simulink model "Week2_pr2"  (R2020b)
settings: Solver=VariableStepAuto  StartTime=0.0  StopTime=10.0  RelTol=1e-3
model workspace (MAT data in the model file):
  Be = 2
  Bv = 1
  Fn = [0  0; 1  0.8; 2  1.6; 3  1.6; 4  1.6; 5  1.6; 6  0.8; 7  0; 8  0; 9  0; 10  0]
  Ie = 1
  Iv = 5
  Muk = 1
  Mus = 1.5
  R = 1
  Tin = [1  2; 2  2; 3  2; 4  2; 5  2; 6  0; 7  0; 8  0; 9  0; 10  0]
settings Model: Creator=user  LastModifiedBy=user

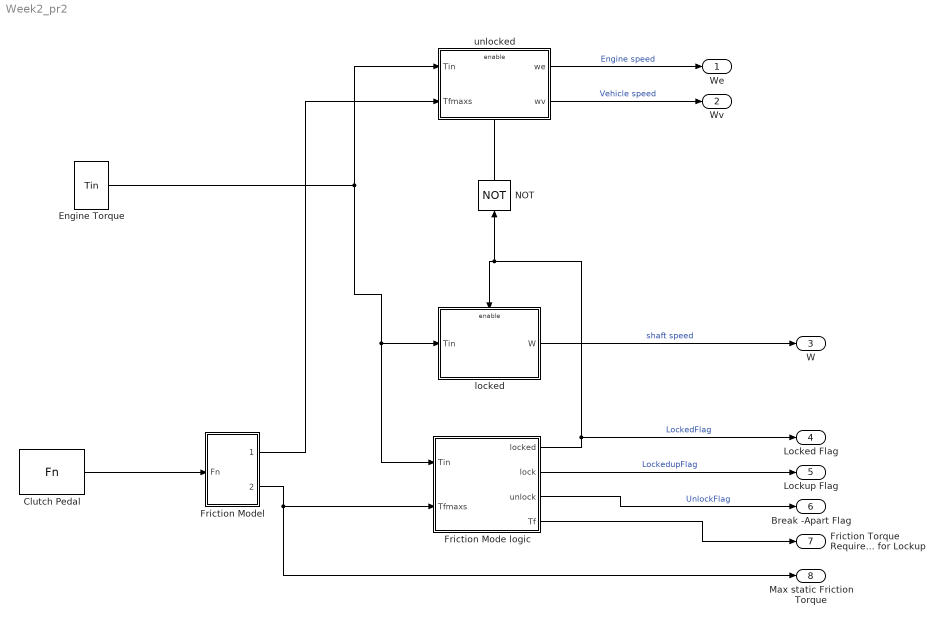
== system Week2_pr2 ==
  Clutch Pedal : FromWorkspace  VariableName=Fn  ZeroCross=off
  Engine Torque : FromWorkspace  VariableName=Tin  ZeroCross=off
  Friction Mode logic : Subsystem
  Friction Model : Subsystem
  NOT : Logic  Operator=NOT  IconShape=distinctive  AllPortsSameDT=off  OutDataTypeStr=fixdt(1,16)
  locked : Subsystem
  unlocked : Subsystem
  We : Outport
  Wv : Outport  Port=2
  W : Outport  Port=3
  Locked Flag : Outport  Port=4
  Lockup Flag : Outport  Port=5
  Break -Apart Flag : Outport  Port=6
  "Friction Torque Required for Lockup " : Outport  Port=7
  Max static Friction Torque : Outport  Port=8
  wires:
  Friction Mode logic/2(lock) -> Lockup Flag/1  "LockedupFlag"
  Friction Model/2(Tfmaxs) -> Max static Friction Torque/1, Friction Mode logic/2(Tfmaxs)
  unlocked/1(we) -> We/1  "Engine speed"
  Friction Mode logic/1(locked) -> Locked Flag/1, NOT/1, locked/Enable  "LockedFlag"
  Friction Mode logic/3(unlock) -> Break -Apart Flag/1  "UnlockFlag"
  locked/1(W) -> W/1  "shaft speed"
  Clutch Pedal/1 -> Friction Model/1(Fn)
  NOT/1 -> unlocked/Enable
  unlocked/2(wv) -> Wv/1  "Vehicle speed"
  Engine Torque/1 -> Friction Mode logic/1(Tin), locked/1(Tin), unlocked/1(Tin)
  Friction Model/1(Tfmaxk) -> unlocked/2(Tfmaxs)
  Friction Mode logic/4(Tf) -> "Friction Torque Required for Lockup "/1

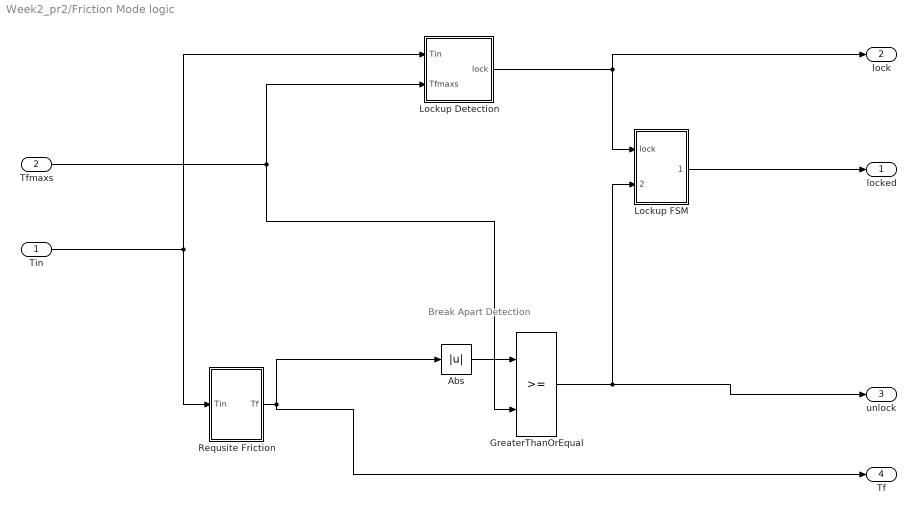
== system Week2_pr2/Friction Mode logic ==
  note: Break Apart Detection
  Tin : Inport
  Tfmaxs : Inport  Port=2
  Abs : Abs
  GreaterThanOrEqual : RelationalOperator  OutDataTypeStr=boolean  RndMeth=Simplest
  Lockup Detection : Subsystem
  Lockup FSM : Subsystem
  Requsite Friction : Subsystem
  locked : Outport
  lock : Outport  Port=2
  unlock : Outport  Port=3
  Tf : Outport  Port=4
  wires:
  Tin/1 -> Requsite Friction/1(Tin), Lockup Detection/1(Tin)
  Lockup FSM/1(locked) -> locked/1
  Lockup Detection/1(lock) -> lock/1, Lockup FSM/1(lock)
  GreaterThanOrEqual/1 -> unlock/1, Lockup FSM/2(unlock)
  Abs/1 -> GreaterThanOrEqual/1
  Tfmaxs/1 -> Lockup Detection/2(Tfmaxs), GreaterThanOrEqual/2
  Requsite Friction/1(Tf) -> Tf/1, Abs/1

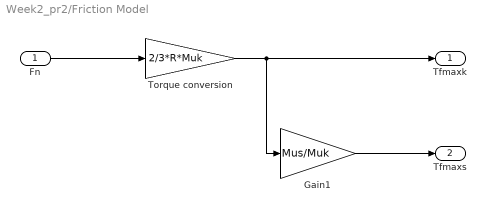
== system Week2_pr2/Friction Model ==
  Fn : Inport
  Gain1 : Gain  Gain=Mus/Muk
  Torque conversion : Gain  Gain=2/3*R*Muk
  Tfmaxk : Outport
  Tfmaxs : Outport  Port=2
  wires:
  Fn/1 -> Torque conversion/1
  Torque conversion/1 -> Gain1/1, Tfmaxk/1
  Gain1/1 -> Tfmaxs/1

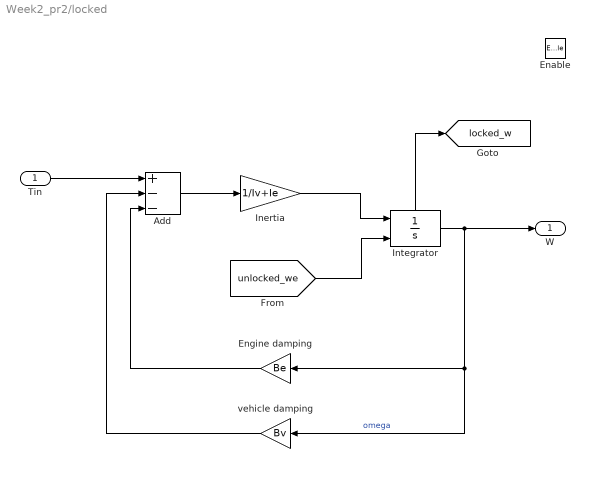
== system Week2_pr2/locked ==
  Tin : Inport
  Enable : EnablePort
  Add : Sum  Inputs=+--
  Engine damping : Gain  Gain=Be
  Inertia : Gain  Gain=1/Iv+Ie
  Integrator : Integrator  InitialConditionSource=external  ShowStatePort=on
  vehicle damping : Gain  Gain=Bv
  W : Outport
  tag scope: locked_w=global
  wires:
  vehicle damping/1 -> Add/2
  Integrator/1 -> W/1, Engine damping/1, vehicle damping/1  "omega"
  Tin/1 -> Add/1
  Engine damping/1 -> Add/3
  Integrator/State -> [locked_w]
  Inertia/1 -> Integrator/1
  Add/1 -> Inertia/1
  [unlocked_we] -> Integrator/2

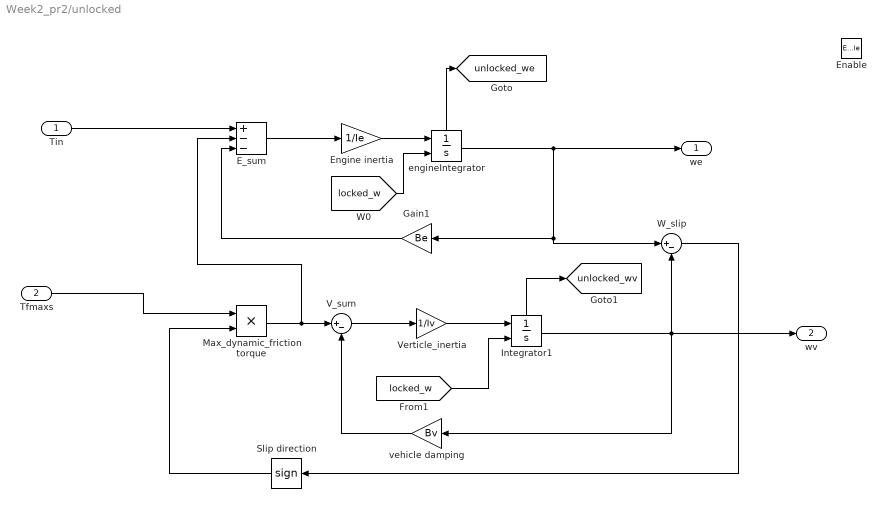
== system Week2_pr2/unlocked ==
  Tin : Inport
  Tfmaxs : Inport  Port=2
  Enable : EnablePort
  E_sum : Sum  Inputs=+--
  Engine inertia : Gain  Gain=1/Ie
  Gain1 : Gain  Gain=Be
  Integrator1 : Integrator  InitialConditionSource=external  ShowStatePort=on
  Max_dynamic_friction torque : Product
  Slip direction : Signum
  V_sum : Sum  Inputs=|+-
  Verticle_inertia : Gain  Gain=1/Iv
  W_slip : Sum  Inputs=|+-
  engineIntegrator : Integrator  InitialConditionSource=external  ShowStatePort=on
  vehicle damping : Gain  Gain=Bv
  we : Outport
  wv : Outport  Port=2
  tag scope: unlocked_we=global, unlocked_wv=global
  wires:
  Max_dynamic_friction torque/1 -> V_sum/1, E_sum/2
  E_sum/1 -> Engine inertia/1
  engineIntegrator/1 -> we/1, W_slip/1, Gain1/1
  engineIntegrator/State -> [unlocked_we]
  Integrator1/1 -> wv/1, vehicle damping/1, W_slip/2
  Verticle_inertia/1 -> Integrator1/1
  Engine inertia/1 -> engineIntegrator/1
  [locked_w] -> engineIntegrator/2
  Slip direction/1 -> Max_dynamic_friction torque/2
  Gain1/1 -> E_sum/3
  [locked_w] -> Integrator1/2
  W_slip/1 -> Slip direction/1
  Integrator1/State -> [unlocked_wv]
  V_sum/1 -> Verticle_inertia/1
  Tin/1 -> E_sum/1
  vehicle damping/1 -> V_sum/2
  Tfmaxs/1 -> Max_dynamic_friction torque/1

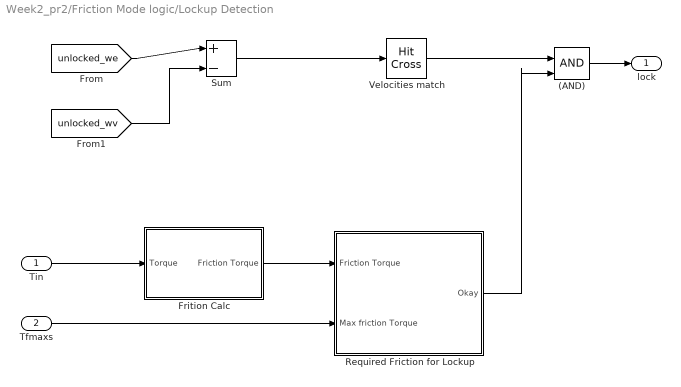
== system Week2_pr2/Friction Mode logic/Lockup Detection ==
  Tin : Inport
  Tfmaxs : Inport  Port=2
  (AND) : Logic  IconShape=distinctive  AllPortsSameDT=off  OutDataTypeStr=boolean
  Frition Calc : Subsystem
  Required Friction for Lockup : Subsystem
  Sum : Sum  Inputs=|+-
  Velocities match : HitCross
  lock : Outport
  wires:
  Tin/1 -> Frition Calc/1(Torque)
  [unlocked_we] -> Sum/1
  [unlocked_wv] -> Sum/2
  Sum/1 -> Velocities match/1
  (AND)/1 -> lock/1
  Frition Calc/1(Friction Torque) -> Required Friction for Lockup/1(Friction Torque)
  Tfmaxs/1 -> Required Friction for Lockup/2(Max friction Torque)
  Required Friction for Lockup/1(Okay) -> (AND)/2
  Velocities match/1 -> (AND)/1

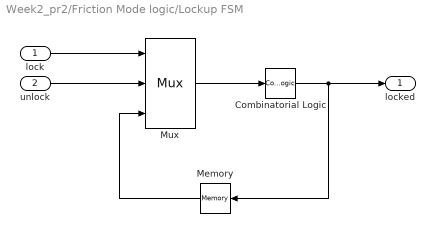
== system Week2_pr2/Friction Mode logic/Lockup FSM ==
  lock : Inport
  unlock : Inport  Port=2
  Combinatorial Logic : CombinatorialLogic  TruthTable=[0;1;0;0;1;1;1;0]
  Memory : Memory
  Mux : Mux  Inputs=3
  locked : Outport
  wires:
  lock/1 -> Mux/1
  unlock/1 -> Mux/2
  Mux/1 -> Combinatorial Logic/1
  Combinatorial Logic/1 -> Memory/1, locked/1
  Memory/1 -> Mux/3

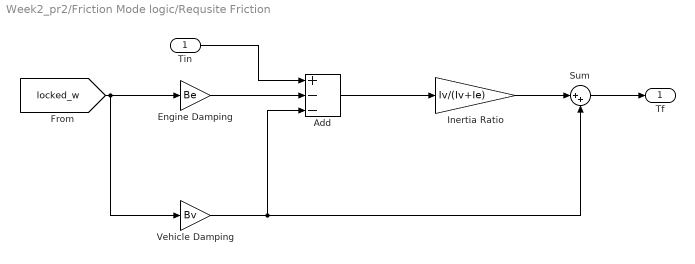
== system Week2_pr2/Friction Mode logic/Requsite Friction ==
  Tin : Inport
  Add : Sum  Inputs=+--
  Engine Damping : Gain  Gain=Be
  Inertia Ratio : Gain  Gain=Iv/(Iv+Ie)
  Sum : Sum  Inputs=|++
  Vehicle Damping : Gain  Gain=Bv
  Tf : Outport
  wires:
  [locked_w] -> Vehicle Damping/1, Engine Damping/1
  Engine Damping/1 -> Add/2
  Vehicle Damping/1 -> Sum/2, Add/3
  Tin/1 -> Add/1
  Add/1 -> Inertia Ratio/1
  Inertia Ratio/1 -> Sum/1
  Sum/1 -> Tf/1

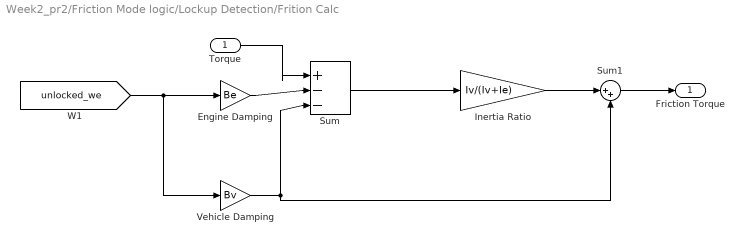
== system Week2_pr2/Friction Mode logic/Lockup Detection/Frition Calc ==
  Torque : Inport
  Engine Damping : Gain  Gain=Be
  Inertia Ratio : Gain  Gain=Iv/(Iv+Ie)
  Sum : Sum  Inputs=|+--
  Sum1 : Sum  Inputs=|++
  Vehicle Damping : Gain  Gain=Bv
  Friction Torque : Outport
  wires:
  [unlocked_we] -> Vehicle Damping/1, Engine Damping/1
  Engine Damping/1 -> Sum/2
  Vehicle Damping/1 -> Sum1/2, Sum/3
  Torque/1 -> Sum/1
  Sum/1 -> Inertia Ratio/1
  Inertia Ratio/1 -> Sum1/1
  Sum1/1 -> Friction Torque/1

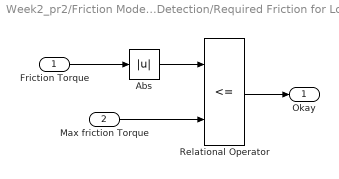
== system Week2_pr2/Friction Mode logic/Lockup Detection/Required Friction for Lockup ==
  Friction Torque : Inport
  Max friction Torque : Inport  Port=2
  Abs : Abs
  Relational Operator : RelationalOperator  Operator=<=  OutDataTypeStr=boolean  RndMeth=Simplest
  Okay : Outport
  wires:
  Friction Torque/1 -> Abs/1
  Max friction Torque/1 -> Relational Operator/2
  Abs/1 -> Relational Operator/1
  Relational Operator/1 -> Okay/1
